simulink model "PCM_DPCM"  (R2016b)
settings: Solver=VariableStepAuto  StartTime=0.0  StopTime=160/2400  RelTol=1e-3
libraries: dsparch4 x7, commsrccod2 x4, commutil2 x4, commchan3 x2
settings Model: Creator=white  LastModifiedBy=white

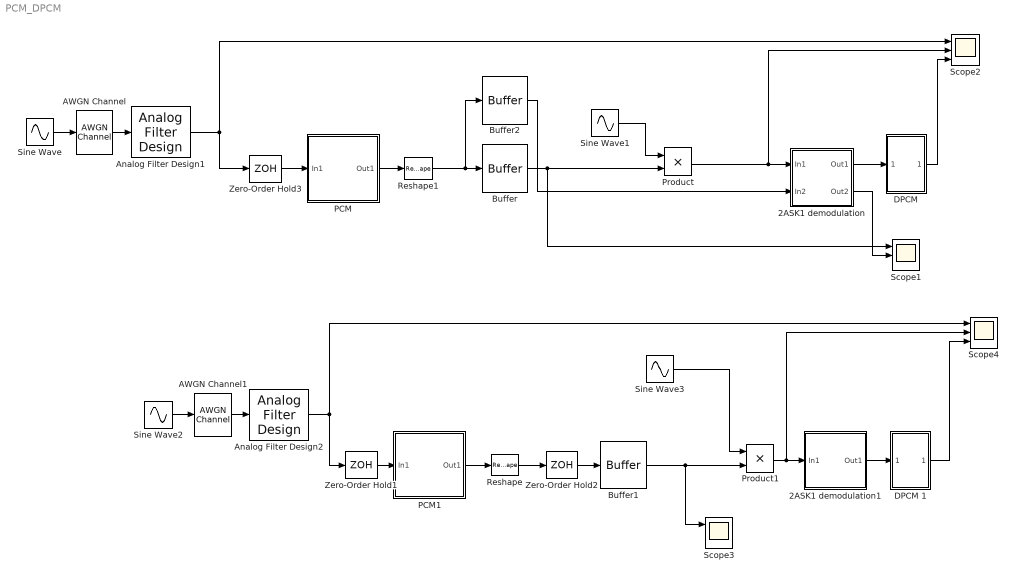
== system PCM_DPCM ==
  2ASK1 demodulation : Subsystem
  2ASK1 demodulation1 : Subsystem
  AWGN Channel : commchan3/AWGN Channel  InputProcessing=Columns as channels (frame based)  seed=67  noiseMode=Variance from mask  EbNodB=10  EsNodB=10  SNRdB=10  bitsPerSym=1  Ps=1  Tsym=1  variance=3
  AWGN Channel1 : commchan3/AWGN Channel  InputProcessing=Columns as channels (frame based)  seed=67  noiseMode=Variance from mask  EbNodB=10  EsNodB=10  SNRdB=10  bitsPerSym=1  Ps=1  Tsym=1  variance=0.01
  Analog Filter Design1 : dsparch4/Analog Filter Design  method=Butterworth  filttype=Lowpass  N=8  Wlo=2*120*pi  Whi=80  Rp=2  Rs=40
  Analog Filter Design2 : dsparch4/Analog Filter Design  method=Butterworth  filttype=Lowpass  N=1  Wlo=2*120*pi  Whi=80  Rp=2  Rs=40
  Buffer : Buffer  N=1  TreatMby1Signals=One channel  OutputFrames=off
  Buffer1 : Buffer  N=1  TreatMby1Signals=One channel  OutputFrames=off
  Buffer2 : Buffer  N=24  TreatMby1Signals=One channel  OutputFrames=off
  "DPCM " : Subsystem
  DPCM 1 : Subsystem
  PCM : Subsystem
  PCM1 : Subsystem
  Product : Product
  Product1 : Product
  Reshape : Reshape
  Reshape1 : Reshape
  Scope{1..4} (4 alike) : Scope  NumInputPorts=3
  Sine Wave : Sin  Amplitude=0.8  Frequency=2*100*pi  SampleTime=1/400
  Sine Wave1 : Sin  Frequency=24000*2*pi  SampleTime=0
  Sine Wave2 : Sin  Frequency=2*100*pi  SampleTime=0
  Sine Wave3 : Sin  Frequency=24000*2*pi  SampleTime=0
  Zero-Order Hold1 : ZeroOrderHold  SampleTime=1/300
  Zero-Order Hold2 : ZeroOrderHold  SampleTime=1/300
  Zero-Order Hold3 : ZeroOrderHold  SampleTime=1/300
  wires:
  AWGN Channel/1 -> Analog Filter Design1/1
  Sine Wave/1 -> AWGN Channel/1
  Analog Filter Design1/1 -> Scope2/1, Zero-Order Hold3/1
  Sine Wave1/1 -> Product/1
  PCM/1(Out1) -> Reshape1/1
  Reshape1/1 -> Buffer2/1, Buffer/1
  Product/1 -> Scope2/2, 2ASK1 demodulation/1(In1)
  "DPCM "/1(Out1) -> Scope2/3
  Buffer/1 -> Product/2, Scope1/1
  AWGN Channel1/1 -> Analog Filter Design2/1
  Sine Wave2/1 -> AWGN Channel1/1
  Analog Filter Design2/1 -> Zero-Order Hold1/1, Scope4/1
  Sine Wave3/1 -> Product1/1
  PCM1/1(Out1) -> Reshape/1
  Reshape/1 -> Zero-Order Hold2/1
  Zero-Order Hold2/1 -> Buffer1/1
  Product1/1 -> Scope4/2, 2ASK1 demodulation1/1(In1)
  2ASK1 demodulation1/1(Out1) -> DPCM 1/1(In1)
  DPCM 1/1(Out1) -> Scope4/3
  Buffer1/1 -> Product1/2, Scope3/1
  Zero-Order Hold3/1 -> PCM/1(In1)
  Zero-Order Hold1/1 -> PCM1/1(In1)
  2ASK1 demodulation/2(Out2) -> Scope1/2
  2ASK1 demodulation/1(Out1) -> "DPCM "/1(In1)
  Buffer2/1 -> 2ASK1 demodulation/2(In2)

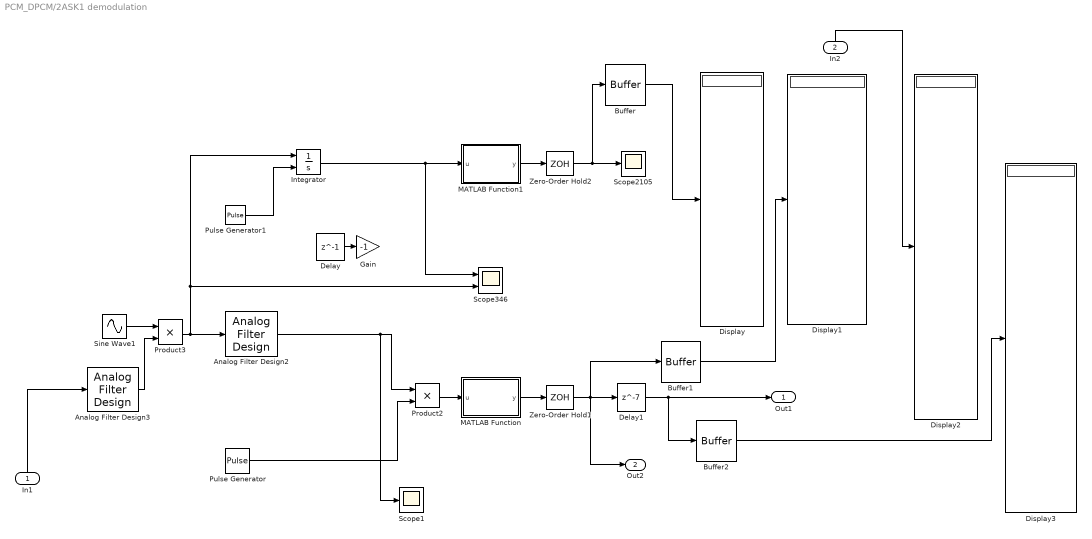
== system PCM_DPCM/2ASK1 demodulation ==
  In1 : Inport
  In2 : Inport  Port=2
  Analog Filter Design2 : dsparch4/Analog Filter Design  method=Butterworth  filttype=Lowpass  N=1  Wlo=800*2*pi  Whi=2*20500*pi  Rp=2  Rs=40
  Analog Filter Design3 : dsparch4/Analog Filter Design  method=Butterworth  filttype=Bandpass  N=1  Wlo=2*21000*pi  Whi=2*27000*pi  Rp=2  Rs=40
  Buffer : Buffer  N=24  TreatMby1Signals=One channel  OutputFrames=off
  Buffer1 : Buffer  N=24  TreatMby1Signals=One channel  OutputFrames=off
  Buffer2 : Buffer  N=24  TreatMby1Signals=One channel  OutputFrames=off
  Delay : Delay  DelayLength=1  InitialCondition=0  SampleTime=1/2400
  Delay1 : Delay  DelayLength=7  InitialCondition=0  SampleTime=1/2400
  Display{,1..3} (4 alike) : Display
  Gain : Gain  Gain=-1
  Integrator : Integrator  ExternalReset=rising
  MATLAB Function : MATLAB Function  TreatAsAtomicUnit=on
  MATLAB Function1 : MATLAB Function  TreatAsAtomicUnit=on
  Product2 : Product
  Product3 : Product
  Pulse Generator : DiscretePulseGenerator  PulseType=Time based  Period=1/2400  PulseWidth=5
  Pulse Generator1 : DiscretePulseGenerator  PulseType=Time based  Period=1/2400  PulseWidth=5  PhaseDelay=1/9600
  Scope1 : Scope
  Scope2105 : Scope
  Scope346 : Scope  NumInputPorts=2
  Sine Wave1 : Sin  Frequency=24000*2*pi  SampleTime=0
  Zero-Order Hold1 : ZeroOrderHold  SampleTime=1/2400
  Zero-Order Hold2 : ZeroOrderHold  SampleTime=1/2400
  Out1 : Outport
  Out2 : Outport  Port=2
  wires:
  In1/1 -> Analog Filter Design3/1
  Analog Filter Design2/1 -> Scope1/1, Product2/1
  Pulse Generator/1 -> Product2/2
  Product2/1 -> MATLAB Function/1(u)
  MATLAB Function/1(y) -> Zero-Order Hold1/1
  Zero-Order Hold2/1 -> Buffer/1, Scope2105/1
  Pulse Generator1/1 -> Integrator/2
  MATLAB Function1/1(y) -> Zero-Order Hold2/1
  Integrator/1 -> Scope346/1, MATLAB Function1/1(u)
  Delay/1 -> Gain/1
  Zero-Order Hold1/1 -> Out2/1, Delay1/1, Buffer1/1
  Sine Wave1/1 -> Product3/1
  Analog Filter Design3/1 -> Product3/2
  Product3/1 -> Integrator/1, Scope346/2, Analog Filter Design2/1
  Buffer/1 -> Display/1
  Buffer1/1 -> Display1/1
  In2/1 -> Display2/1
  Delay1/1 -> Buffer2/1, Out1/1
  Buffer2/1 -> Display3/1

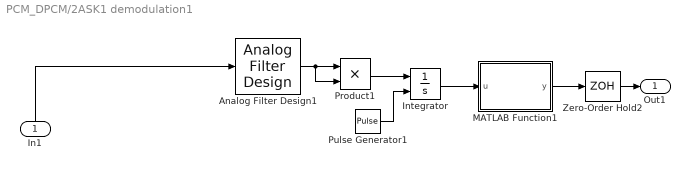
== system PCM_DPCM/2ASK1 demodulation1 ==
  In1 : Inport
  Analog Filter Design1 : dsparch4/Analog Filter Design  method=Butterworth  filttype=Bandpass  N=1  Wlo=2*23500*pi  Whi=2*24500*pi  Rp=2  Rs=40
  Integrator : Integrator  ExternalReset=rising
  MATLAB Function1 : MATLAB Function  TreatAsAtomicUnit=on
  Product1 : Product
  Pulse Generator1 : DiscretePulseGenerator  PulseType=Time based  Period=1/800  PulseWidth=5  PhaseDelay=1/1600
  Zero-Order Hold2 : ZeroOrderHold  SampleTime=1/800
  Out1 : Outport
  wires:
  Zero-Order Hold2/1 -> Out1/1
  Analog Filter Design1/1 -> Product1/2, Product1/1
  Product1/1 -> Integrator/1
  Pulse Generator1/1 -> Integrator/2
  MATLAB Function1/1(y) -> Zero-Order Hold2/1
  Integrator/1 -> MATLAB Function1/1(u)
  In1/1 -> Analog Filter Design1/1

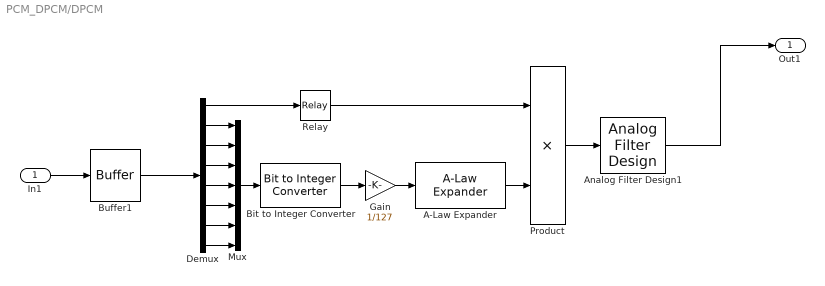
== system PCM_DPCM/DPCM  ==
  In1 : Inport
  A-Law Expander : commsrccod2/A-Law Expander  A=87.6  V=1
  Analog Filter Design1 : dsparch4/Analog Filter Design  method=Butterworth  filttype=Lowpass  N=8  Wlo=2*120*pi  Whi=80  Rp=2  Rs=40
  Bit to Integer Converter : commutil2/Bit to Integer Converter  nbits=7  bitOrder=MSB first  signedOutputValues=Unsigned  outDtype=Inherit via internal rule  outDtypeSigned=Inherit via internal rule
  Buffer1 : Buffer  N=8  TreatMby1Signals=One channel  OutputFrames=off
  Demux : Demux  Outputs=8
  Gain : Gain  Gain=1/127
  Mux : Mux  Inputs=7
  Product : Product
  Relay : Relay  OnSwitchValue=0.5  OffSwitchValue=0.5  OnOutputValue=-1  OffOutputValue=1
  Out1 : Outport
  wires:
  Demux/2 -> Mux/1
  Demux/3 -> Mux/2
  Demux/4 -> Mux/3
  Demux/5 -> Mux/4
  Demux/6 -> Mux/5
  Demux/7 -> Mux/6
  Demux/8 -> Mux/7
  Bit to Integer Converter/1 -> Gain/1
  Mux/1 -> Bit to Integer Converter/1
  Relay/1 -> Product/1
  Gain/1 -> A-Law Expander/1
  Demux/1 -> Relay/1
  A-Law Expander/1 -> Product/2
  Buffer1/1 -> Demux/1
  Product/1 -> Analog Filter Design1/1
  In1/1 -> Buffer1/1
  Analog Filter Design1/1 -> Out1/1

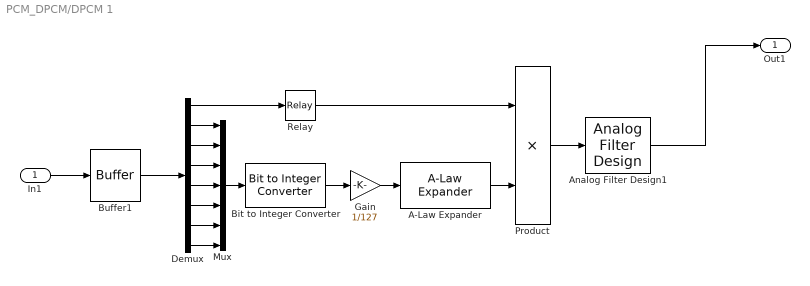
== system PCM_DPCM/DPCM 1 ==
  In1 : Inport
  A-Law Expander : commsrccod2/A-Law Expander  A=87.6  V=1
  Analog Filter Design1 : dsparch4/Analog Filter Design  method=Butterworth  filttype=Lowpass  N=8  Wlo=2*120*pi  Whi=80  Rp=2  Rs=40
  Bit to Integer Converter : commutil2/Bit to Integer Converter  nbits=7  bitOrder=MSB first  signedOutputValues=Unsigned  outDtype=Inherit via internal rule  outDtypeSigned=Inherit via internal rule
  Buffer1 : Buffer  N=8  TreatMby1Signals=One channel  OutputFrames=off
  Demux : Demux  Outputs=8
  Gain : Gain  Gain=1/127
  Mux : Mux  Inputs=7
  Product : Product
  Relay : Relay  OnSwitchValue=0.5  OffSwitchValue=0.5  OnOutputValue=-1  OffOutputValue=1
  Out1 : Outport
  wires:
  Demux/2 -> Mux/1
  Demux/3 -> Mux/2
  Demux/4 -> Mux/3
  Demux/5 -> Mux/4
  Demux/6 -> Mux/5
  Demux/7 -> Mux/6
  Demux/8 -> Mux/7
  Bit to Integer Converter/1 -> Gain/1
  Mux/1 -> Bit to Integer Converter/1
  Relay/1 -> Product/1
  Gain/1 -> A-Law Expander/1
  Demux/1 -> Relay/1
  A-Law Expander/1 -> Product/2
  Buffer1/1 -> Demux/1
  Product/1 -> Analog Filter Design1/1
  In1/1 -> Buffer1/1
  Analog Filter Design1/1 -> Out1/1

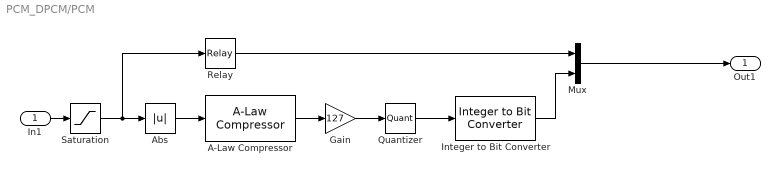
== system PCM_DPCM/PCM ==
  In1 : Inport
  A-Law Compressor : commsrccod2/A-Law Compressor  A=87.6  V=1
  Abs : Abs
  Gain : Gain  Gain=127
  Integer to Bit Converter : commutil2/Integer to Bit Converter  nbits=7  signedInputValues=Unsigned  bitOrder=MSB first  outDtype=Inherit via internal rule
  Mux : Mux  Inputs=2
  Quantizer : Quantizer  QuantizationInterval=1
  Relay : Relay  OnSwitchValue=0  OffSwitchValue=0  OnOutputValue=0  OffOutputValue=1
  Saturation : Saturate  UpperLimit=1  LowerLimit=-1
  Out1 : Outport
  wires:
  In1/1 -> Saturation/1
  Abs/1 -> A-Law Compressor/1
  A-Law Compressor/1 -> Gain/1
  Integer to Bit Converter/1 -> Mux/2
  Gain/1 -> Quantizer/1
  Relay/1 -> Mux/1
  Quantizer/1 -> Integer to Bit Converter/1
  Saturation/1 -> Relay/1, Abs/1
  Mux/1 -> Out1/1

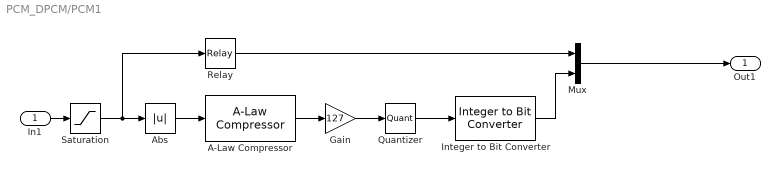
== system PCM_DPCM/PCM1 ==
  In1 : Inport
  A-Law Compressor : commsrccod2/A-Law Compressor  A=87.6  V=1
  Abs : Abs
  Gain : Gain  Gain=127
  Integer to Bit Converter : commutil2/Integer to Bit Converter  nbits=7  signedInputValues=Unsigned  bitOrder=MSB first  outDtype=Inherit via internal rule
  Mux : Mux  Inputs=2
  Quantizer : Quantizer  QuantizationInterval=1
  Relay : Relay  OnSwitchValue=0  OffSwitchValue=0  OnOutputValue=0  OffOutputValue=1
  Saturation : Saturate  UpperLimit=1  LowerLimit=-1
  Out1 : Outport
  wires:
  In1/1 -> Saturation/1
  Abs/1 -> A-Law Compressor/1
  A-Law Compressor/1 -> Gain/1
  Integer to Bit Converter/1 -> Mux/2
  Gain/1 -> Quantizer/1
  Relay/1 -> Mux/1
  Quantizer/1 -> Integer to Bit Converter/1
  Saturation/1 -> Relay/1, Abs/1
  Mux/1 -> Out1/1

== matlab function PCM_DPCM/2ASK1 demodulation/MATLAB Function1 ==
  data: u input; y output
function y = fcn(u)
if(u>0.0001)
    u=1
else
    u=0
end
y = u;

== matlab function PCM_DPCM/2ASK1 demodulation1/MATLAB Function1 ==
  data: u input; y output
function y = fcn(u)
if(u>0.0002)
    u=1
else
    u=0
end
y = u;

== matlab function PCM_DPCM/2ASK1 demodulation/MATLAB Function ==
  data: u input; y output
function y = fcn(u)
if(u>0.25)
    u=1
else
    u=0
end
y = u;
